simulink model "dororo_global"  (R2024b)
settings: Solver=FixedStepAuto  StartTime=0.0  StopTime=150  FixedStep=0.01  RelTol=1e-3
PreLoadFcn:
  | start_loc = [5,5,0];
  | goal_loc = [95,95,0];
model workspace (MAT data in the model file):
  initial_yaw = 0
undefined symbols (not defined in the file or in its folder): map
libraries: autolibshared x1, slpidlib x1
settings Model: Creator=1155t  LastModifiedBy=l
settings DataIOCC: SaveFormat=Array  ReturnWorkspaceOutputs=off
settings RTWCC: GPUComputeCapability=3.5

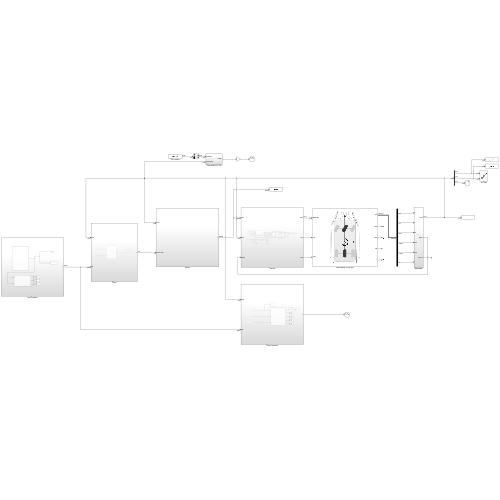
[thumbnail: Simulink's stored preview of the top-level diagram]
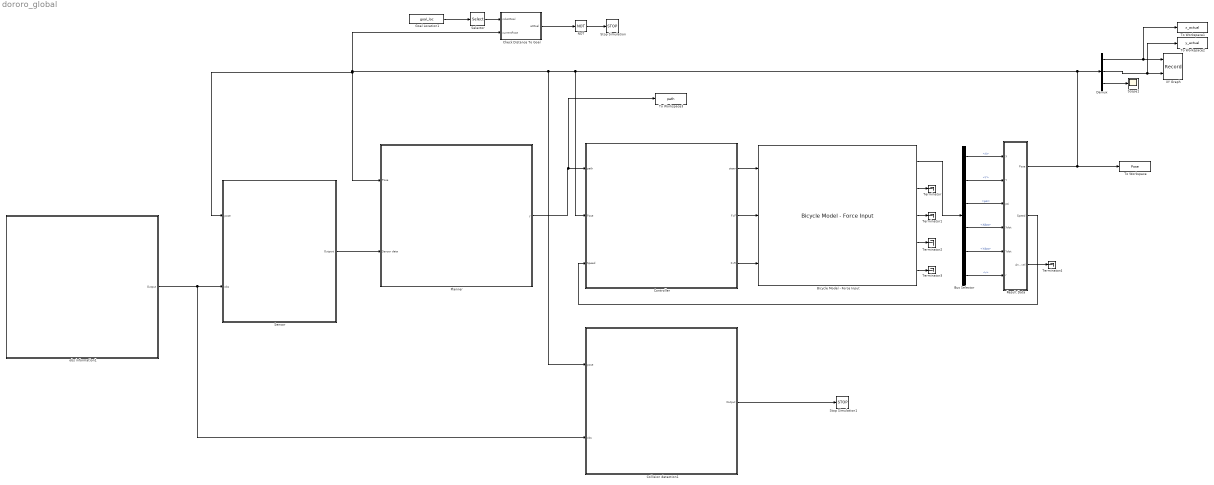
== system dororo_global ==
  Bicycle Model - Force Input : autolibshared/Bicycle Model - Force Input  trackMode=Single (bicycle)  inputMode=External longitudinal forces  frontSteerMode=on  rearSteerMode=off  windMode=off  muMode=off  extFMode=off  extMMode=off  aMode=3  NF=2  NR=2  m=2000  a=1.5  b=1.5  h=0.75  X_o=start_loc(1)  xdot_o=0  CalphaMode=off  sigmaMode=on  w=[1.4,1.4]  Cy_f=12e3  Cy_r=11e3  sigma_f=.1  sigma_r=.1  alpha_f_brk=[-.1 .1]  Cy_f_data=[-9e3 9e3]  alpha_r_brk=[-.1 .1]  Cy_r_data=[-9e3 9e3]  Y_o=start_loc(2)  ydot_o=0  Izz=4000  psi_o=0  r_o=0  Af=2  Cd=.3  Cl=.1  Cpm=.1  beta_w=[0 0.01:0.01:0.3]  Cs=[0 0.01:0.01:0.3]  Cym=[0 1e-6:0.01:0.3]  Pabs=101325  Tair=273  g=9.81  mu=1  xdot_tol=.01  Fznom=5000  Fxtire_sat=1e6  Fytire_sat=1e6  longOff=0  latOff=0  vertOff=0
      settings: LibrarySourceBlock=drivingscenarioandsensors/Bicycle Model - Force Input
  Bus Selector : BusSelector  OutputSignals=InertFrm.Cg.Disp.X,InertFrm.Cg.Disp.Y,InertFrm.Cg.Ang.psi,InertFrm.Cg.Vel.Xdot,InertFrm.Cg.Vel.Ydot,BdyFrm.Cg.AngVel.r
  Check Distance To Goal : Subsystem
  Collision detection1 : Subsystem
  Controller : Subsystem
  Demux : Demux  Outputs=3
  Goal Location1 : Constant  Value=goal_loc  VectorParams1D=off
  NOT : Logic  Operator=NOT  IconShape=distinctive  AllPortsSameDT=off  OutDataTypeStr=boolean
  Planner : Subsystem
  Result Data : Subsystem
  Scope1 : Scope
  Selector : Selector  InputPortWidth=3  IndexOptions=Index vector (dialog)  Indices=[1 2]  OutputSizes=1
  Sensor : Subsystem
  Stop Simulation : Stop
  Stop Simulation1 : Stop
  Terminator{,1..4} (5 alike) : Terminator
  To Workspace : ToWorkspace  VariableName=Pose  SampleTime=-1
  To Workspace1 : ToWorkspace  VariableName=x_actual  SaveFormat=Timeseries  SampleTime=-1
  To Workspace2 : ToWorkspace  VariableName=y_actual  SaveFormat=Timeseries  SampleTime=-1
  To Workspace3 : ToWorkspace  VariableName=path  SaveFormat=Timeseries  SampleTime=-1
  XY Graph : Record  FileSettingsInternal="{\"entries\":[{\"content\":{\"excelSettings\":{\"content\":{},\"type\":\"Streamout.ExcelSettings\"}},\"type\":\"Streamout.FileSettingStorage\",\"uuid\":\"\"}],\"packageUris\":[\"http:\\/\\/schema.mathworks.com\\/mf0\\/streamout_blocks\\/R2020a\"],\"version\":\"1.0\"}"  Layout=[1 1]  SignalsInternal="{\"entries\":[{\"content\":{\"signals\":[{\"content\":{\"blockPath\":[],\"dimensions\":[1,1],\"domain\":\"\",\"lineColor\":\"#fe330a\",\"lineWidth\":2,\"plots\":[ 1 ],\"port\":1,\"sid\":[\"\"],\"signalID\":1,\"signalName\":\"Demux:1\"},\"type\":\"RecordBlkView.Signal\",\"uuid\":\"\"},{\"content\":{\"blockPath\":[],\"dimensions\":[1,1],\"domain\":\"\",\"lineColor\":\"#22b573\",\"lineWidth\":2,\"plots\":[ 1 ],\"port\":2,\"sid\":[\"\"],\"signalID\":2,\"signalName\":\"Demux:2\"},\"type\":\"RecordBlkView.Signal\",\"uuid\":\"\"}]},\"type\":\"RecordBlkView.InputSignals\",\"uuid\":\"\"}],\"packageUris\":[\"http:\\/\\/schema.mathworks.com\\/mf0\\/streamout_blocks\\/R2020a\"],\"version\":\"1.0\"}"  VisualizationBindings="{\"xyplotplugin\":{\"info\":[{\"series\":[{\"bindingParametersList\":[{\"parameter\":\"X-Axis\",\"signalID\":1,\"signalName\":\"Demux:1\"},{\"parameter\":\"Y-Axis\",\"signalID\":2,\"signalName\":\"Demux:2\"}],\"seriesID\":0}],\"subplotID\":1}]}}"  CompatibilityTag=XY
  obs information1 : Subsystem
  wires:
  Check Distance To Goal/1(atGoal) -> NOT/1
  NOT/1 -> Stop Simulation/1
  Demux/1 -> To Workspace1/1, XY Graph/1
  Demux/2 -> To Workspace2/1, XY Graph/2
  Result Data/1(Pose) -> To Workspace/1, Controller/2(Pose), Collision detection1/1(pose), Check Distance To Goal/2(currentPose), Sensor/1(pose), Planner/1("Pose "), Demux/1
  Collision detection1/1(Output) -> Stop Simulation1/1
  Selector/1 -> Check Distance To Goal/1(robotGoal)
  Goal Location1/1 -> Selector/1
  obs information1/1(Output) -> Collision detection1/2(obs), Sensor/2(obs)
  Demux/3 -> Scope1/1
  Bicycle Model - Force Input/1 -> Bus Selector/1
  Controller/1(steer) -> Bicycle Model - Force Input/1
  Controller/2(FxF) -> Bicycle Model - Force Input/2
  Controller/3(FxR) -> Bicycle Model - Force Input/3
  Bus Selector/1 -> Result Data/1(X)  "<X>"
  Bus Selector/2 -> Result Data/2(Y)  "<Y>"
  Bus Selector/3 -> Result Data/3(psi)  "<psi>"
  Bus Selector/4 -> Result Data/4(Xdot)  "<Xdot>"
  Bus Selector/5 -> Result Data/5(Ydot)  "<Ydot>"
  Bus Selector/6 -> Result Data/6(r)  "<r>"
  Bicycle Model - Force Input/2 -> Terminator/1
  Bicycle Model - Force Input/3 -> Terminator1/1
  Bicycle Model - Force Input/4 -> Terminator2/1
  Bicycle Model - Force Input/5 -> Terminator3/1
  Sensor/1(Outport) -> Planner/2(Sensor data)
  Planner/1(y) -> To Workspace3/1, Controller/1(path)
  Result Data/2(Speed) -> Controller/3(Speed)
  Result Data/3(Ang_vel) -> Terminator4/1

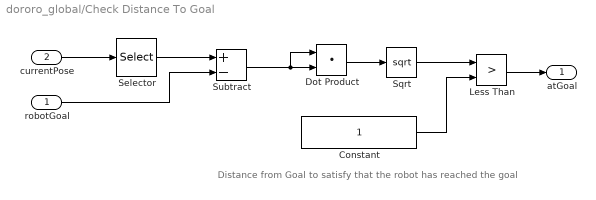
== system dororo_global/Check Distance To Goal ==
  note: Distance from Goal to satisfy that the robot has reached the goal
  robotGoal : Inport
  currentPose : Inport  Port=2
  Constant : Constant
  Dot Product : DotProduct  OutDataTypeStr=Inherit: Inherit via internal rule
  Less Than : RelationalOperator  Operator=>  OutDataTypeStr=boolean  RndMeth=Simplest  InputSameDT=off
  Selector : Selector  InputPortWidth=3  IndexOptions=Index vector (dialog)  Indices=[1 2]  OutputSizes=1
  Sqrt : Sqrt
  Subtract : Sum  Inputs=+-
  atGoal : Outport
  wires:
  robotGoal/1 -> Subtract/2
  Dot Product/1 -> Sqrt/1
  Constant/1 -> Less Than/2
  currentPose/1 -> Selector/1
  Less Than/1 -> atGoal/1
  Sqrt/1 -> Less Than/1
  Subtract/1 -> Dot Product/1, Dot Product/2
  Selector/1 -> Subtract/1

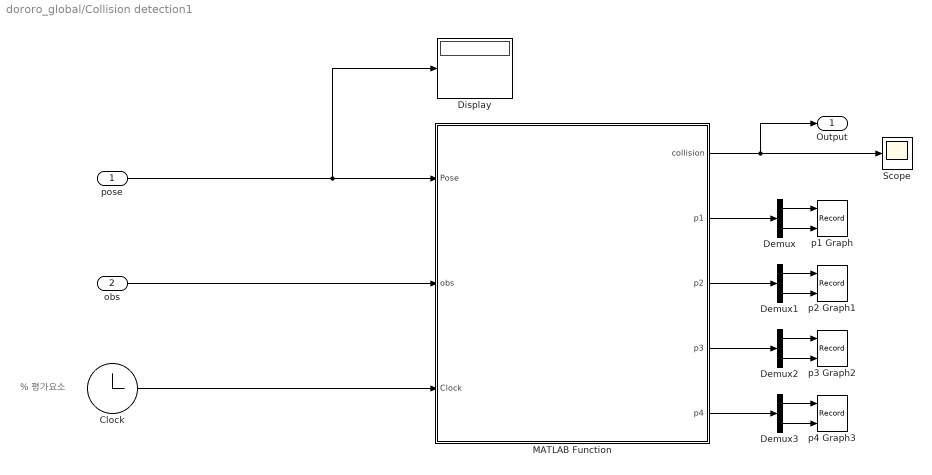
== system dororo_global/Collision detection1 ==
  note: % 평가요소
  pose : Inport
  obs : Inport  Port=2
  Clock : Clock
  Demux{,1..3} (4 alike) : Demux  Outputs=2
  Display : Display
  MATLAB Function : MATLAB Function  TreatAsAtomicUnit=on
  Scope : Scope
  p1 Graph : Record  FileSettingsInternal="{\"entries\":[{\"content\":{\"excelSettings\":{\"content\":{},\"type\":\"Streamout.ExcelSettings\"}},\"type\":\"Streamout.FileSettingStorage\",\"uuid\":\"\"}],\"packageUris\":[\"http:\\/\\/schema.mathworks.com\\/mf0\\/streamout_blocks\\/R2020a\"],\"version\":\"1.0\"}"  Layout=[1 1]  SignalsInternal="{\"entries\":[{\"content\":{\"signals\":[{\"content\":{\"blockPath\":[],\"dimensions\":[1,1],\"domain\":\"\",\"lineColor\":\"#64d413\",\"lineWidth\":2,\"port\":1,\"sid\":[\"\"],\"signalID\":1,\"signalName\":\"Demux:1\"},\"type\":\"RecordBlkView.Signal\",\"uuid\":\"\"},{\"content\":{\"blockPath\":[],\"dimensions\":[1,1],\"domain\":\"\",\"lineColor\":\"#ff13a6\",\"lineWidth\":2,\"port\":2,\"sid\":[\"\"],\"signalID\":2,\"signalName\":\"Demux:2\"},\"type\":\"RecordBlkView.Signal\",\"uuid\":\"\"}]},\"type\":\"RecordBlkView.InputSignals\",\"uuid\":\"\"}],\"packageUris\":[\"http:\\/\\/schema.mathworks.com\\/mf0\\/streamout_blocks\\/R2020a\"],\"version\":\"1.0\"}"  VisualizationBindings="{\"xyplotplugin\":{\"info\":[{\"series\":[],\"subplotID\":1}]}}"  CompatibilityTag=XY
  p2 Graph1 : Record  FileSettingsInternal="{\"entries\":[{\"content\":{\"excelSettings\":{\"content\":{},\"type\":\"Streamout.ExcelSettings\"}},\"type\":\"Streamout.FileSettingStorage\",\"uuid\":\"\"}],\"packageUris\":[\"http:\\/\\/schema.mathworks.com\\/mf0\\/streamout_blocks\\/R2020a\"],\"version\":\"1.0\"}"  Layout=[1 1]  SignalsInternal="{\"entries\":[{\"content\":{\"signals\":[{\"content\":{\"blockPath\":[],\"dimensions\":[1,1],\"domain\":\"\",\"lineColor\":\"#fe330a\",\"lineWidth\":2,\"port\":1,\"sid\":[\"\"],\"signalID\":1,\"signalName\":\"Demux1:1\"},\"type\":\"RecordBlkView.Signal\",\"uuid\":\"\"},{\"content\":{\"blockPath\":[],\"dimensions\":[1,1],\"domain\":\"\",\"lineColor\":\"#22b573\",\"lineWidth\":2,\"port\":2,\"sid\":[\"\"],\"signalID\":2,\"signalName\":\"Demux1:2\"},\"type\":\"RecordBlkView.Signal\",\"uuid\":\"\"}]},\"type\":\"RecordBlkView.InputSignals\",\"uuid\":\"\"}],\"packageUris\":[\"http:\\/\\/schema.mathworks.com\\/mf0\\/streamout_blocks\\/R2020a\"],\"version\":\"1.0\"}"  VisualizationBindings="{\"xyplotplugin\":{\"info\":[{\"series\":[],\"subplotID\":1}]}}"  CompatibilityTag=XY
  p3 Graph2 : Record  FileSettingsInternal="{\"entries\":[{\"content\":{\"excelSettings\":{\"content\":{},\"type\":\"Streamout.ExcelSettings\"}},\"type\":\"Streamout.FileSettingStorage\",\"uuid\":\"\"}],\"packageUris\":[\"http:\\/\\/schema.mathworks.com\\/mf0\\/streamout_blocks\\/R2020a\"],\"version\":\"1.0\"}"  Layout=[1 1]  SignalsInternal="{\"entries\":[{\"content\":{\"signals\":[{\"content\":{\"blockPath\":[],\"dimensions\":[1,1],\"domain\":\"\",\"lineColor\":\"#0072bd\",\"lineWidth\":2,\"port\":1,\"sid\":[\"\"],\"signalID\":1,\"signalName\":\"Demux2:1\"},\"type\":\"RecordBlkView.Signal\",\"uuid\":\"\"},{\"content\":{\"blockPath\":[],\"dimensions\":[1,1],\"domain\":\"\",\"lineColor\":\"#d95319\",\"lineWidth\":2,\"port\":2,\"sid\":[\"\"],\"signalID\":2,\"signalName\":\"Demux2:2\"},\"type\":\"RecordBlkView.Signal\",\"uuid\":\"\"}]},\"type\":\"RecordBlkView.InputSignals\",\"uuid\":\"\"}],\"packageUris\":[\"http:\\/\\/schema.mathworks.com\\/mf0\\/streamout_blocks\\/R2020a\"],\"version\":\"1.0\"}"  VisualizationBindings="{\"xyplotplugin\":{\"info\":[{\"series\":[],\"subplotID\":1}]}}"  CompatibilityTag=XY
  p4 Graph3 : Record  FileSettingsInternal="{\"entries\":[{\"content\":{\"excelSettings\":{\"content\":{},\"type\":\"Streamout.ExcelSettings\"}},\"type\":\"Streamout.FileSettingStorage\",\"uuid\":\"\"}],\"packageUris\":[\"http:\\/\\/schema.mathworks.com\\/mf0\\/streamout_blocks\\/R2020a\"],\"version\":\"1.0\"}"  Layout=[1 1]  SignalsInternal="{\"entries\":[{\"content\":{\"signals\":[{\"content\":{\"blockPath\":[],\"dimensions\":[1,1],\"domain\":\"\",\"lineColor\":\"#edb120\",\"lineWidth\":2,\"port\":1,\"sid\":[\"\"],\"signalID\":1,\"signalName\":\"Demux3:1\"},\"type\":\"RecordBlkView.Signal\",\"uuid\":\"\"},{\"content\":{\"blockPath\":[],\"dimensions\":[1,1],\"domain\":\"\",\"lineColor\":\"#7e2f8e\",\"lineWidth\":2,\"port\":2,\"sid\":[\"\"],\"signalID\":2,\"signalName\":\"Demux3:2\"},\"type\":\"RecordBlkView.Signal\",\"uuid\":\"\"}]},\"type\":\"RecordBlkView.InputSignals\",\"uuid\":\"\"}],\"packageUris\":[\"http:\\/\\/schema.mathworks.com\\/mf0\\/streamout_blocks\\/R2020a\"],\"version\":\"1.0\"}"  VisualizationBindings="{\"xyplotplugin\":{\"info\":[{\"series\":[],\"subplotID\":1}]}}"  CompatibilityTag=XY
  Output : Outport
  wires:
  pose/1 -> Display/1, MATLAB Function/1(Pose)
  Clock/1 -> MATLAB Function/3(Clock)
  obs/1 -> MATLAB Function/2(obs)
  MATLAB Function/1(collision) -> Output/1, Scope/1
  MATLAB Function/2(p1) -> Demux/1
  Demux/1 -> p1 Graph/1
  Demux/2 -> p1 Graph/2
  Demux1/2 -> p2 Graph1/2
  MATLAB Function/3(p2) -> Demux1/1
  Demux1/1 -> p2 Graph1/1
  Demux2/2 -> p3 Graph2/2
  MATLAB Function/4(p3) -> Demux2/1
  Demux2/1 -> p3 Graph2/1
  Demux3/2 -> p4 Graph3/2
  MATLAB Function/5(p4) -> Demux3/1
  Demux3/1 -> p4 Graph3/1

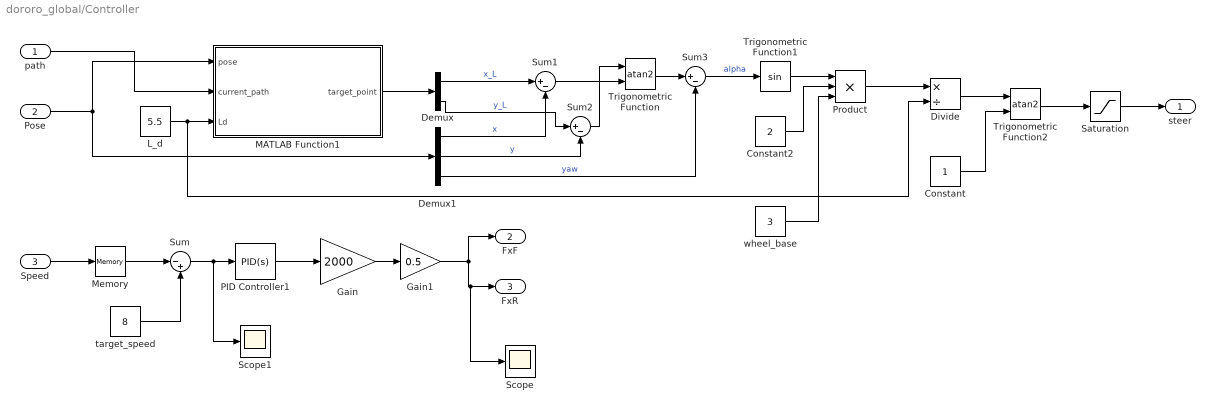
== system dororo_global/Controller ==
  path : Inport
  Pose : Inport  Port=2
  Speed : Inport  Port=3
  Constant : Constant
  Constant2 : Constant  Value=2
  Demux : Demux  Outputs=2
  Demux1 : Demux  Outputs=3
  Divide : Product  Inputs=*/
  Gain : Gain  Gain=2000
  Gain1 : Gain  Gain=0.5
  L_d : Constant  Value=5.5
  MATLAB Function1 : MATLAB Function  TreatAsAtomicUnit=on
  Memory : Memory
  PID Controller1 : slpidlib/PID Controller  Controller=PID  Form=Parallel  TimeDomain=Continuous-time  UseExternalTs=off  SampleTime=-1  IntegratorMethod=Forward Euler  FilterMethod=Forward Euler  ControllerParametersSource=internal  P=2.5  I=0.1  UseKiTs=off  D=0.05  UseExternalDerivativeSource=off  N=100  UseFilter=on  TunerSelectOption=Transfer Function Based (PID Tuner App)  InitialConditionSource=internal  InitialConditionForIntegrator=0  InitialConditionForFilter=0  DifferentiatorICPrevScaledInput=0  ExternalReset=none  TrackingMode=off  Kt=1  LimitOutput=off  SatLimitsSource=internal  UpperSaturationLimit=inf  LowerSaturationLimit=-inf  LinearizeAsGain=on  AntiWindupMode=none  Kb=1  LimitIntegrator=off  UpperIntegratorSaturationLimit=inf  LowerIntegratorSaturationLimit=-inf  POutMin=[]  POutMax=[]  IOutMin=[]  IOutMax=[]  DOutMin=[]  DOutMax=[]  NOutMin=[]  NOutMax=[]  SumOutMin=[]  SumOutMax=[]  SaturationOutMin=[]  SaturationOutMax=[]  PParamMin=[]  PParamMax=[]  IParamMin=[]  IParamMax=[]  DParamMin=[]  DParamMax=[]  NParamMin=[]  NParamMax=[]  KbParamMin=[]  KbParamMax=[]  KtParamMin=[]  KtParamMax=[]  KbOutMin=[]  KbOutMax=[]  KtOutMin=[]  KtOutMax=[]  IntegratorOutMin=[]  IntegratorOutMax=[]  FilterOutMin=[]  FilterOutMax=[]  SumI1OutMin=[]  SumI1OutMax=[]  SumI2OutMin=[]  SumI2OutMax=[]  SumI3OutMin=[]  SumI3OutMax=[]  SumI4OutMin=[]  SumI4OutMax=[]  SumDOutMin=[]  SumDOutMax=[]  DifferentiatorOutMin=[]  DifferentiatorOutMax=[]  FilterDiffOutCoefMin=[]  FilterDiffOutCoefMax=[]  ReciprocalOutMin=[]  ReciprocalOutMax=[]  SumDenOutMin=[]  SumDenOutMax=[]  SumNumOutMin=[]  SumNumOutMax=[]  DivideOutMin=[]  DivideOutMax=[]  UdiffTsProdOutMin=[]  UdiffTsProdOutMax=[]  NTsProdOutMin=[]  NTsProdOutMax=[]  UintegralTsProdOutMin=[]  UintegralTsProdOutMax=[]  UngainTsProdOutMin=[]  UngainTsProdOutMax=[]  ClampingZeroOutDataTypeStr=Inherit: Inherit via back propagation  ClampingZeroOutMin=[]  ClampingZeroOutMax=[]  FilterDenConstantOutDataTypeStr=Inherit: Inherit via back propagation  FilterDenConstantOutMin=[]  FilterDenConstantOutMax=[]  PCopyOutDataTypeStr=Inherit: Inherit via back propagation  PCopyOutMin=[]  PCopyOutMax=[]  NCopyOutDataTypeStr=Inherit: Inherit via back propagation  NCopyOutMin=[]  NCopyOutMax=[]  IntegratorContinuousStateAttributes=''  IntegratorStateMustResolveToSignalObject=off  IntegratorRTWStateStorageClass=Auto  FilterContinuousStateAttributes=''  FilterStateMustResolveToSignalObject=off  FilterRTWStateStorageClass=Auto  ParallelPVariant=InternalParameters  IdealPVariant=Disabled  IVariant=InternalParameters  DVariant=InternalParameters  IntegratorVariant=Continuous  SatVariant=Disabled  AWVariant=Passthrough  PCopyVariant=Disabled  TRVariant=Disabled  FdbkBlocksVariant=Forward  IdealPFdbkVariant=Disabled  SatFdbkVariant=Disabled  DerivativeFilterVariant=ContFilter  NVariant=InternalParameters  NCopyVariant=Disabled  FilterICVariant=InternalICsFilter  IntegratorICVariant=InternalICs  ExternalResetVariant=Disabled  TRSumVariant=Passthrough  SumFdbkVariant=Disabled  SumVariant=Sum_PID  TsampFilterVariant=InternalTs  TsampNgainVariant=Passthrough  TsampIntegralVariant=Disabled_SignalSpec  ExternalSaturationOutDataTypeStr=Inherit: Same as second input  DerivativeSourceVariant=ErrorSignal  PreIntVariant=InternalPreInt
  Product : Product  Inputs=3
  Saturation : Saturate  UpperLimit=pi/4  LowerLimit=-pi/4
  Scope : Scope
  Scope1 : Scope
  Sum : Sum  Inputs=|-+
  Sum1 : Sum  Inputs=|+-
  Sum2 : Sum  Inputs=|+-
  Sum3 : Sum  Inputs=|+-
  Trigonometric Function : Trigonometry  Operator=atan2
  Trigonometric Function1 : Trigonometry
  Trigonometric Function2 : Trigonometry  Operator=atan2
  target_speed : Constant  Value=8
  wheel_base : Constant  Value=3
  steer : Outport
  FxF : Outport  Port=2
  FxR : Outport  Port=3
  wires:
  path/1 -> MATLAB Function1/2(current_path)
  Pose/1 -> Demux1/1, MATLAB Function1/1(pose)
  target_speed/1 -> Sum/2
  PID Controller1/1 -> Gain/1
  Sum/1 -> Scope1/1, PID Controller1/1
  Gain/1 -> Gain1/1
  Gain1/1 -> Scope/1, FxR/1, FxF/1
  L_d/1 -> Divide/2, MATLAB Function1/3(Ld)
  MATLAB Function1/1(target_point) -> Demux/1
  Demux1/1 -> Sum1/2  "x"
  Demux1/2 -> Sum2/2  "y"
  Demux/2 -> Sum2/1  "y_L"
  Demux/1 -> Sum1/1  "x_L"
  Demux1/3 -> Sum3/2  "yaw"
  Sum1/1 -> Trigonometric Function/2
  Sum2/1 -> Trigonometric Function/1
  Trigonometric Function/1 -> Sum3/1
  Sum3/1 -> Trigonometric Function1/1  "alpha"
  Trigonometric Function1/1 -> Product/1
  Constant2/1 -> Product/2
  wheel_base/1 -> Product/3
  Product/1 -> Divide/1
  Trigonometric Function2/1 -> Saturation/1
  Speed/1 -> Memory/1
  Divide/1 -> Trigonometric Function2/1
  Constant/1 -> Trigonometric Function2/2
  Saturation/1 -> steer/1
  Memory/1 -> Sum/1

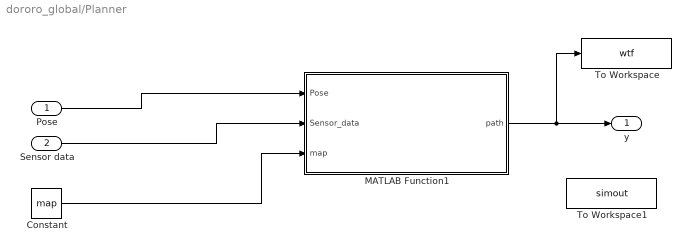
== system dororo_global/Planner ==
  "Pose " : Inport
  Sensor data : Inport  Port=2
  Constant : Constant  Value=map
  MATLAB Function1 : MATLAB Function  TreatAsAtomicUnit=on
  To Workspace : ToWorkspace  VariableName=wtf  SaveFormat=Timeseries  SampleTime=-1
  To Workspace1 : ToWorkspace  VariableName=simout  SaveFormat=Timeseries  SampleTime=-1
  y : Outport
  wires:
  Sensor data/1 -> MATLAB Function1/2(Sensor_data)
  "Pose "/1 -> MATLAB Function1/1(Pose)
  MATLAB Function1/1(path) -> To Workspace/1, y/1
  Constant/1 -> MATLAB Function1/3(map)

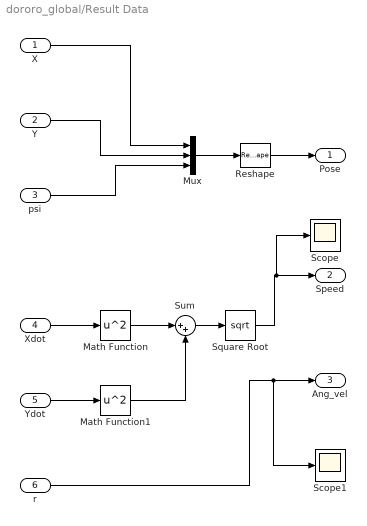
== system dororo_global/Result Data ==
  X : Inport
  Y : Inport  Port=2
  psi : Inport  Port=3
  Xdot : Inport  Port=4
  Ydot : Inport  Port=5
  r : Inport  Port=6
  Math Function : Math  Operator=square
  Math Function1 : Math  Operator=square
  Mux : Mux  Inputs=3
  Reshape : Reshape  OutputDimensionality=Row vector (2-D)
  Scope : Scope
  Scope1 : Scope
  Square Root : Sqrt
  Sum : Sum  Inputs=|++
  Pose : Outport
  Speed : Outport  Port=2
  Ang_vel : Outport  Port=3
  wires:
  Mux/1 -> Reshape/1
  X/1 -> Mux/1
  Y/1 -> Mux/2
  psi/1 -> Mux/3
  Xdot/1 -> Math Function/1
  Ydot/1 -> Math Function1/1
  Math Function/1 -> Sum/1
  Math Function1/1 -> Sum/2
  Sum/1 -> Square Root/1
  Square Root/1 -> Scope/1, Speed/1
  r/1 -> Scope1/1, Ang_vel/1
  Reshape/1 -> Pose/1

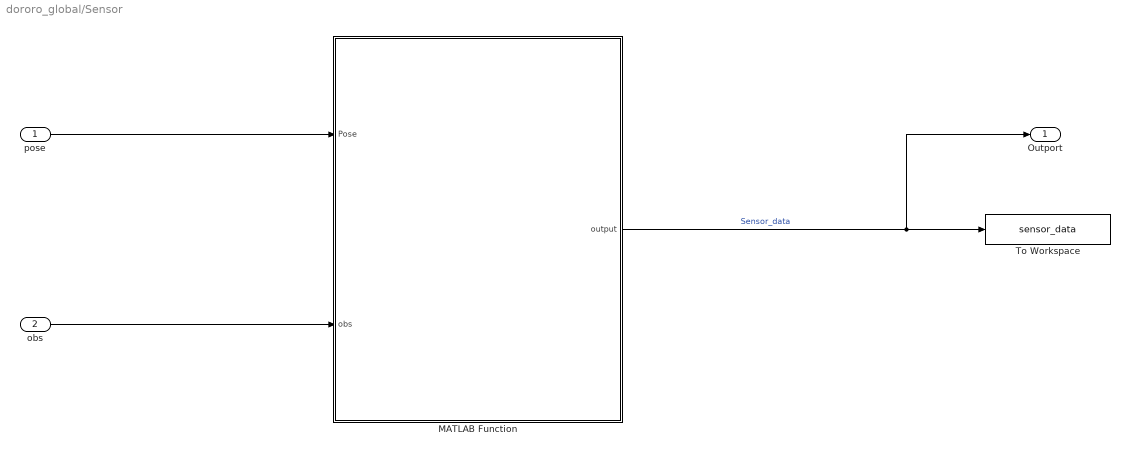
== system dororo_global/Sensor ==
  pose : Inport
  obs : Inport  Port=2
  MATLAB Function : MATLAB Function  TreatAsAtomicUnit=on
  To Workspace : ToWorkspace  VariableName=sensor_data  SampleTime=-1
  Outport : Outport
  wires:
  pose/1 -> MATLAB Function/1(Pose)
  obs/1 -> MATLAB Function/2(obs)
  MATLAB Function/1(output) -> Outport/1, To Workspace/1  "Sensor_data"

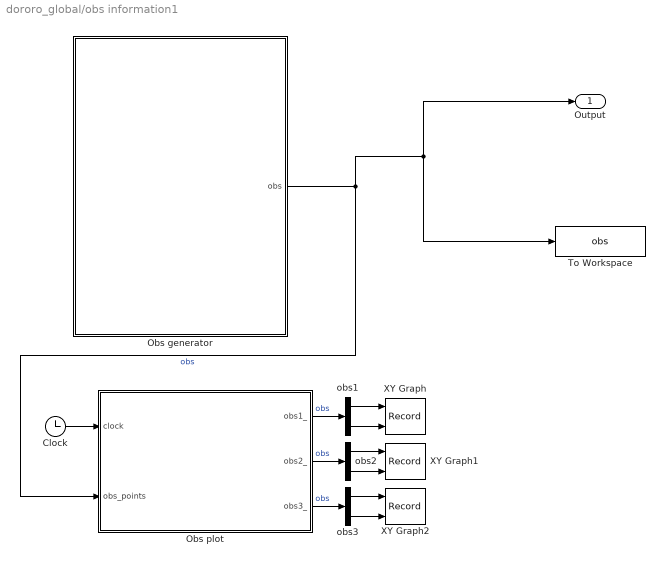
== system dororo_global/obs information1 ==
  Clock : Clock
  Obs generator : MATLAB Function  TreatAsAtomicUnit=on
  Obs plot : MATLAB Function  TreatAsAtomicUnit=on
  To Workspace : ToWorkspace  VariableName=obs  SampleTime=-1
  XY Graph : Record  FileSettingsInternal="{\"entries\":[{\"content\":{\"excelSettings\":{\"content\":{},\"type\":\"Streamout.ExcelSettings\"}},\"type\":\"Streamout.FileSettingStorage\",\"uuid\":\"\"}],\"packageUris\":[\"http:\\/\\/schema.mathworks.com\\/mf0\\/streamout_blocks\\/R2020a\"],\"version\":\"1.0\"}"  Layout=[1 1]  SignalsInternal="{\"entries\":[{\"content\":{\"signals\":[{\"content\":{\"blockPath\":[],\"dimensions\":[1,1],\"domain\":\"\",\"lineColor\":\"#0072bd\",\"lineWidth\":2,\"port\":1,\"sid\":[\"\"],\"signalID\":1,\"signalName\":\"obs1:1\"},\"type\":\"RecordBlkView.Signal\",\"uuid\":\"\"},{\"content\":{\"blockPath\":[],\"dimensions\":[1,1],\"domain\":\"\",\"lineColor\":\"#d95319\",\"lineWidth\":2,\"port\":2,\"sid\":[\"\"],\"signalID\":2,\"signalName\":\"obs1:2\"},\"type\":\"RecordBlkView.Signal\",\"uuid\":\"\"}]},\"type\":\"RecordBlkView.InputSignals\",\"uuid\":\"\"}],\"packageUris\":[\"http:\\/\\/schema.mathworks.com\\/mf0\\/streamout_blocks\\/R2020a\"],\"version\":\"1.0\"}"  VisualizationBindings="{\"xyplotplugin\":{\"info\":[{\"series\":[],\"subplotID\":1}]}}"  CompatibilityTag=XY
  XY Graph1 : Record  FileSettingsInternal="{\"entries\":[{\"content\":{\"excelSettings\":{\"content\":{},\"type\":\"Streamout.ExcelSettings\"}},\"type\":\"Streamout.FileSettingStorage\",\"uuid\":\"\"}],\"packageUris\":[\"http:\\/\\/schema.mathworks.com\\/mf0\\/streamout_blocks\\/R2020a\"],\"version\":\"1.0\"}"  Layout=[1 1]  SignalsInternal="{\"entries\":[{\"content\":{\"signals\":[{\"content\":{\"blockPath\":[],\"dimensions\":[1,1],\"domain\":\"\",\"lineColor\":\"#edb120\",\"lineWidth\":2,\"port\":1,\"sid\":[\"\"],\"signalID\":1,\"signalName\":\"obs2:1\"},\"type\":\"RecordBlkView.Signal\",\"uuid\":\"\"},{\"content\":{\"blockPath\":[],\"dimensions\":[1,1],\"domain\":\"\",\"lineColor\":\"#7e2f8e\",\"lineWidth\":2,\"port\":2,\"sid\":[\"\"],\"signalID\":2,\"signalName\":\"obs2:2\"},\"type\":\"RecordBlkView.Signal\",\"uuid\":\"\"}]},\"type\":\"RecordBlkView.InputSignals\",\"uuid\":\"\"}],\"packageUris\":[\"http:\\/\\/schema.mathworks.com\\/mf0\\/streamout_blocks\\/R2020a\"],\"version\":\"1.0\"}"  VisualizationBindings="{\"xyplotplugin\":{\"info\":[{\"series\":[],\"subplotID\":1}]}}"  CompatibilityTag=XY
  XY Graph2 : Record  FileSettingsInternal="{\"entries\":[{\"content\":{\"excelSettings\":{\"content\":{},\"type\":\"Streamout.ExcelSettings\"}},\"type\":\"Streamout.FileSettingStorage\",\"uuid\":\"\"}],\"packageUris\":[\"http:\\/\\/schema.mathworks.com\\/mf0\\/streamout_blocks\\/R2020a\"],\"version\":\"1.0\"}"  Layout=[1 1]  SignalsInternal="{\"entries\":[{\"content\":{\"signals\":[{\"content\":{\"blockPath\":[],\"dimensions\":[1,1],\"domain\":\"\",\"lineColor\":\"#77ac30\",\"lineWidth\":2,\"port\":1,\"sid\":[\"\"],\"signalID\":1,\"signalName\":\"obs3:1\"},\"type\":\"RecordBlkView.Signal\",\"uuid\":\"\"},{\"content\":{\"blockPath\":[],\"dimensions\":[1,1],\"domain\":\"\",\"lineColor\":\"#4dbeee\",\"lineWidth\":2,\"port\":2,\"sid\":[\"\"],\"signalID\":2,\"signalName\":\"obs3:2\"},\"type\":\"RecordBlkView.Signal\",\"uuid\":\"\"}]},\"type\":\"RecordBlkView.InputSignals\",\"uuid\":\"\"}],\"packageUris\":[\"http:\\/\\/schema.mathworks.com\\/mf0\\/streamout_blocks\\/R2020a\"],\"version\":\"1.0\"}"  VisualizationBindings="{\"xyplotplugin\":{\"info\":[{\"series\":[],\"subplotID\":1}]}}"  CompatibilityTag=XY
  obs1 : Demux  Outputs=2
  obs2 : Demux  Outputs=2
  obs3 : Demux  Outputs=2
  Output : Outport
  wires:
  Obs generator/1(obs) -> To Workspace/1, Output/1, Obs plot/2(obs_points)  "obs"
  obs2/2 -> XY Graph1/2
  obs1/2 -> XY Graph/2
  Obs plot/2(obs2_) -> obs2/1  "obs"
  Clock/1 -> Obs plot/1(clock)
  obs2/1 -> XY Graph1/1
  Obs plot/1(obs1_) -> obs1/1  "obs"
  obs3/2 -> XY Graph2/2
  obs1/1 -> XY Graph/1
  Obs plot/3(obs3_) -> obs3/1  "obs"
  obs3/1 -> XY Graph2/1

== matlab function dororo_global/Sensor/MATLAB Function ==
  settings: updateMethod=CONTINUOUS  sampleTime=0.01
  data: output output size=120; Pose input; obs input
function output = Sensor(Pose,obs)

%-----------------<Release Information >----------------------------
% version: alpha 1.0.0 (For distribution)
% Release Date: 2023.11.11
% Developer: Yu su Hyung
%-------------------------------------------------------------------

% <Block Description>
% The block was created to generate sensor data from the vehicle's current location and obstacle information. 
% Use a function called Inpolygon to find the distance between the obstruction and the vehicle.
% You can adjust the resolution and visibility of the sensor.

% Warning!!
% This algorithm calculates the sensor distance from the number of points within the obstacle area, 
% which can lead to errors if the sensor distance is longer than the thickness of the obstacle.
% 2023.11.6 It is resolved!!

% There may be additional changes depending on the difficulty or progress of the map.

resolution_deg = 120;
sensor_dist = 15;

output = ones(resolution_deg, 1) * sensor_dist;
scan_range = linspace(-60*pi/180, 60*pi/180, resolution_deg);

for output_idx = 1:resolution_deg
    
    scan_angle = scan_range(output_idx);
    d = laser_dist(Pose, sensor_dist, scan_angle, obs);
    output(output_idx) = d;
end

end




function d = dist(q1,q2)
d = sqrt( (q1(1) - q2(1))^2 + ( q1(2) - q2(2))^2 );
end


function [min_laser_dist_, check_block] = laser_dist(pose, sensor_dist, sensor_heading, obs)

% pose: 차량의 현재 위치(x,y,psi)
% sensor_dist: 센서의 가시거리
% sensor_heading: 센서의 방향(현재 차량 header 기준)


check_block = 0;
p0 = [pose(1), pose(2)];
heading = pose(3);

pf = [p0(1) + sensor_dist*cos(heading+sensor_heading), p0(2) + sensor_dist*sin(heading+sensor_heading)];

resolution_dis = 100;
xq = linspace(p0(1), pf(1), resolution_dis);
yq = linspace(p0(2), pf(2), resolution_dis);

min_laser_dist_ = sensor_dist; %default 값

for i = 1: size(obs,1)
    %p1은 왼쪽 상단 점, p2는 오른쪽 하단 점을 의미
    p1_x= obs(i,1);
    p1_y= obs(i,2);
    p2_x= obs(i,3);
    p2_y= obs(i,4);
    
    % obstacle 좌표 -> 시계방향
    xv = [p1_x, p1_x, p2_x, p2_x,p1_x];
    yv = [p1_y, p2_y, p2_y, p1_y,p1_y];
    
    [in,on] = inpolygon(xq,yq,xv,yv);

    for k = 1: size(in,2)
        if in(1, k) ~= 0
            % 장애물 영역 안에 들어가는 좌표 검사
            crossing_x = xq(k);
            crossing_y = yq(k);
            temp = dist([crossing_x, crossing_y], [p0(1), p0(2)]);
        else
            temp = sensor_dist;      
        end

        if temp < min_laser_dist_
            % 센서 최대거리 15m 및 센서 조향각 이내에 장애물이 존재하는 경우    
            min_laser_dist_ = temp;
        end
        
    end   

end

end

== matlab function dororo_global/Planner/MATLAB Function1 ==
  data: path output; Pose input; Sensor_data input; map input
function path = main(Pose, Sensor_data, map)
    % A* Algorithm
    % 1. 초기 설정
    [rows, cols] = size(map);
    max_path_size = 200; % 경로 배열의 최대 크기
    path = NaN(max_path_size, 2); % 최종 경로 출력 변수

    % start & goal
    start = [5, 5];   
    goal = [95, 95];  

    % A* 알고리즘에 필요한 변수 초기화
    visited = false(rows, cols);     % 방문한 노드를 기록하는 배열
    cost = Inf(rows, cols);          % 각 노드까지의 g(n) 비용
    parent = NaN(rows, cols, 2);   % 각 노드의 부모 노드를 기록하는 배열

    cost(start(1), start(2)) = 0;    % 시작점의 g(n) 비용은 0

    % Open list 초기화
    max_open_size = rows * cols;
    open_list = NaN(max_open_size, 3); % [row, col, f_cost]
    open_count = 0;

    h_cost = heuristic(start, goal); % 시작점에서 목표점까지의 휴리스틱 비용 계산 -> 이거 왜?
    open_count = open_count + 1;
    open_list(open_count, :) = [start, cost(start(1), start(2)) + h_cost];

    goal_found = false;

    % 2. 메인 루프 (Main Loop)
    while open_count > 0
        % Open 리스트에서 f_cost가 가장 작은 노드 찾기
        [~, idx] = min(open_list(1:open_count, 3));
        current_node = open_list(idx, 1:2);

        % 찾은 노드를 Open 리스트에서 제거
        open_list(idx, :) = open_list(open_count, :);
        open_count = open_count - 1;

        % 목표점에 도달했는지 확인
        if all(current_node == goal)
            goal_found = true;
            break;
        end

        % 방문 표시
        if visited(current_node(1), current_node(2))
            continue;
        end
        visited(current_node(1), current_node(2)) = true;

        % 이웃 노드 탐색
        neighbors = get_neighbors(current_node, rows, cols);

        for i = 1:size(neighbors, 1)
            neighbor = neighbors(i, :);
            r = neighbor(1);
            c = neighbor(2);

            % 장애물이거나 이미 방문했는지
            if map(r, c) ~= 0 || visited(r,c)
                continue;
            end

            % 현재 노드를 거쳐 이웃 노드로 가는 새로운 g_cost 계산
            move_cost = norm(current_node - neighbor); % 1 또는 sqrt(2)
            g_cost = cost(current_node(1), current_node(2)) + move_cost;

            % 더 나은 경로를 발견했을 때 정보 업데이트
            if g_cost < cost(r, c)
                cost(r, c) = g_cost;
                parent(r, c, :) = current_node;

                % f_cost 계산 및 Open 리스트에 추가
                f_cost = g_cost + heuristic(neighbor, goal);

                open_count = open_count + 1;
                open_list(open_count, :) = [neighbor, f_cost];
            end
        end
    end

    % 3. 경로 역추적 
    if goal_found
        % 경로를 역순으로 추적
        path_temp = goal;
        p_node = goal;

        while ~all(p_node == start)
            parent_node = squeeze(parent(p_node(1), p_node(2), :))';
            path_temp = [parent_node; path_temp];
            p_node = parent_node;
        end

        num_path_points = size(path_temp, 1);
        path(1:num_path_points, :) = path_temp;
        path = path(:, [2, 1])
    end
end

% 휴리스틱 함수 - 유클리드 거리
function h = heuristic(pos, goal)
    h = norm(pos - goal);
end

% 이웃 노드 탐색 함수 
function neighbors = get_neighbors(pos, max_row, max_col)
    neighbors = zeros(8, 2);
    neighbor_count = 0;

    % 8방향 탐색
    directions = [-1, 0; 1, 0; 0, -1; 0, 1; -1, 1; -1, -1; 1, -1; 1, 1];

    for i = 1:8
        r = pos(1) + directions(i, 1);
        c = pos(2) + directions(i, 2);

        % 맵 경계 내에 있는지 확인
        if r >= 1 && r <= max_row && c >= 1 && c <= max_col
            neighbor_count = neighbor_count + 1;
            neighbors(neighbor_count, :) = [r, c];
        end
    end
end

== matlab function dororo_global/Collision detection1/MATLAB Function ==
  settings: updateMethod=CONTINUOUS  sampleTime=0.01
  data: collision output; Pose input; obs input; Clock input; p1 output; p2 output; p3 output; p4 output
function [collision, p1, p2, p3, p4] = fcn(Pose, obs, Clock)

%-----------------<Release Information >----------------------------
% version: alpha 1.0.0 (For distribution)
% Release Date: 2023.11.11
% Developer: You su Hyung
%-------------------------------------------------------------------

%<Block Description>
% This is a block that determines whether there is a collision between the vehicle and an obstacle.
% If the vehicle collides with an obstacle, the simulation ends immediately.
% You don't have to worry about this part.

% Car Information
% 전장: 3m
% 축간 거리: 2.5m
% 전폭: 1.5m

w = 3;
h = 1.5;
resolution = 5; % 충돌 해상도

collision = 0;

p0 = [Pose(1), Pose(2)];
heading = Pose(3); %rad

rotation_mat = [ cos(heading), -sin(heading); sin(heading), cos(heading)]; %roation matrix

p1 = rotation_mat * [- w/2; + h/2 ] + [p0(1); p0(2)]; % rot * 왼쪽 상단 + center
p2 = rotation_mat * [+ w/2; + h/2 ] + [p0(1); p0(2)]; % rot * 오른쪽 상단 + center
p3 = rotation_mat * [+ w/2; - h/2 ] + [p0(1); p0(2)]; % rot * 오른쪽 하단 + center
p4 = rotation_mat * [- w/2; - h/2 ] + [p0(1); p0(2)]; % rot * 왼쪽 하단 + center

xq = [linspace(p1(1), p2(1), resolution), linspace(p2(1), p3(1), resolution), linspace(p3(1), p4(1), resolution), linspace(p4(1), p1(1), resolution) ];
yq = [linspace(p1(2), p2(2), resolution), linspace(p2(2), p3(2), resolution), linspace(p3(2), p4(2), resolution), linspace(p4(2), p1(2), resolution) ];

for i = 1: size(obs,1)
    %p1은 왼쪽 상단 점, p2는 오른쪽 하단 점을 의미
    p1_x= obs(i,1);
    p1_y= obs(i,2);
    p2_x= obs(i,3); 
    p2_y= obs(i,4); 
    
    xv = [p1_x, p1_x, p2_x, p2_x];
    yv = [p1_y, p2_y, p2_y, p1_y];
    
    [in,on] = inpolygon(xq,yq,xv,yv);
    
    n = numel(xq(~in)); %검출점 개수(직사각형 장애물 밖에 있는 점의 개수)
    
    if n ~= 20
        % 외부 점이 20개 이하면 충돌 판단
        collision = 1;
        break;
    else
        collision = 0;
        
    end
end

end

== matlab function dororo_global/Controller/MATLAB Function1 ==
  data: pose input; target_point output; current_path input; Ld input
% function target_point = find_target_point(pose, path, Ld)
%     x = pose(1); y = pose(2);
%     x_path = path(:,2); 
%     y_path = path(:,1);
%     dists = sqrt((x_path-x).^2 + (y_path-y).^2);
%     [~, idx] = min(dists);
% 
%     target_idx = idx;
%     N = size(path,1);
%     while target_idx < N
%         if sqrt((x_path(target_idx)-x)^2 + (y_path(target_idx)-y)^2) >= Ld
%             break;
%         end
%         target_idx = target_idx + 1;
%     end
%     target_point = [x_path(target_idx), y_path(target_idx)];
% end

% function target_point = find_target_point(pose, current_path, Ld)
%
% 입력:
%   pose: 현재 차량의 [x, y, yaw] 벡터
%   current_path: '현재 시간'의 99x2 경로 데이터 (2차원 행렬)
%   Ld: 전방 주시 거리
%
function target_point = find_target_point_corrected(pose, current_path, Ld)
    
    % 현재 차량 위치
    x_vehicle = pose(1);
    y_vehicle = pose(2);

    % --- 문제점 1 수정 ---
    % 경로의 X, Y 좌표를 올바르게 할당
    x_path = current_path(:,1);
    y_path = current_path(:,2);

    % 차량에서 경로의 각 점까지의 거리 계산
    dists = sqrt((x_path - x_vehicle).^2 + (y_path - y_vehicle).^2);

    % 차량과 가장 가까운 경로 점의 인덱스 찾기
    [~, closest_idx] = min(dists);

    % 가장 가까운 점에서부터 Ld 이상 떨어진 목표점 탐색 시작
    target_idx = closest_idx;
    num_path_points = size(current_path,1);

    while target_idx < num_path_points
        dist_to_target = sqrt((x_path(target_idx) - x_vehicle)^2 + (y_path(target_idx) - y_vehicle)^2);
        
        % 차량으로부터의 직선 거리가 Ld를 넘으면 해당 점을 목표점으로 선택
        if dist_to_target >= Ld
            break;
        end
        target_idx = target_idx + 1;
    end
    
    % 최종 목표점 반환
    target_point = [x_path(target_idx), y_path(target_idx)];
end

== matlab function dororo_global/obs information1/Obs generator ==
  settings: updateMethod=DISCRETE
  data: obs output size=[20 4]
function obs = obstacle()

%-----------------<Release Information >----------------------------
% version: alpha 1.0.0 (For distribution)
% Release Date: 2023.11.11
% Developer: You su Hyung
%-------------------------------------------------------------------

%<Block Description>
% This block was created to create obstacles and boundary walls in the map.
% Each obstacle information consists of two points (upper left point and lower right point) and has a size of nx4.
% Obstacle information created in this block is utilized in the impact detection block, the sensor block.

obs = [ 
   0, 100, 100, 98;     % 1
   0, 2, 100, 0;
   0, 98, 2, 2;
   98, 98, 100, 2; 

   12, 70, 98, 68;      % 5
   70, 98, 72, 80;
   20, 68, 44, 54;
   2, 40, 58, 38;
   58, 52, 88, 50;
   58, 50, 60, 25;
   86, 50, 88, 12;
   72, 39, 86, 37;
   32, 28, 34, 2;       % 13
   44, 28, 46, 13;
   46, 15, 60, 13;
   58, 13, 60, 2;
   72, 27, 74, 2;

   22, 82, 28, 72 ;
   36, 96, 42, 86 ;
   47, 80, 53, 70 ;

   ];

% obs = [
%     0, 100, 100, 98;     
%     0, 2, 100, 0;
%     0, 98, 2, 2;
%     98, 98, 100, 2; ];

== matlab function dororo_global/obs information1/Obs plot ==
  settings: updateMethod=DISCRETE
  data: obs1_ output size=[1 2]; obs2_ output size=[1 2]; obs3_ output size=[1 2]; clock input; obs_points input
function [obs1_, obs2_, obs3_] = obstacle(clock, obs_points)

%-----------------<Release Information >----------------------------
% version: alpha 1.0.0 (For distribution)
% Release Date: 2023.11.11
% Developer: You su Hyung
%-------------------------------------------------------------------

%<Block Description>
% This block was created to create obstacles and boundary walls in the map.
% Each obstacle information consists of two points (upper left point and lower right point) and has a size of nx4.
% Obstacle information created in this block is utilized in the impact detection block, the sensor block.

if (clock > 5)
clock = 5;
end

X = 1 + fix(rem(clock, 4));

height = 10;
width = 6;

obs1 = [ 
   obs_points(end-2,1), obs_points(end-2,2); 
   obs_points(end-2,1), obs_points(end-2,2) - height; 
   obs_points(end-2,1)+width, obs_points(end-2,2) - height;
   obs_points(end-2,1)+width, obs_points(end-2,2);];

obs2 = [ 
   obs_points(end-1,1), obs_points(end-1,2); 
   obs_points(end-1,1), obs_points(end-1,2) - height; 
   obs_points(end-1,1)+width, obs_points(end-1,2) - height;
   obs_points(end-1,1)+width, obs_points(end-1,2);];

obs3 = [ 
   obs_points(end,1), obs_points(end,2); 
   obs_points(end,1), obs_points(end,2) - height; 
   obs_points(end,1)+width, obs_points(end,2) - height;
   obs_points(end,1)+width, obs_points(end,2);];

obs1_ = obs1(X,:);
obs2_ = obs2(X,:);
obs3_ = obs3(X,:);




% obs = [
%     0, 100, 100, 98;     
%     0, 2, 100, 0;
%     0, 98, 2, 2;
%     98, 98, 100, 2; ];
